simulink model "with_torque_vectoring"  (R2024b)
settings: Solver=VariableStepAuto  StartTime=0.0  StopTime=10.0  MaxStep=0.001  RelTol=1e-3
values from neighbouring files (symbols this model uses):
  c_yf = 15714    [vehicle_input_data.m]
  c_yr = 21429    [vehicle_input_data.m]
  delta = 1.04    [vehicle_input_data.m]
  dt = 0.001    [vehicle_input_data.m]
  Izz = 120    [vehicle_input_data.m]
  l_f = 0.873    [vehicle_input_data.m]
  l_r = 0.717    [vehicle_input_data.m]
  m = 356    [vehicle_input_data.m]
  VCG = 25    [vehicle_input_data.m]
libraries: slpidlib x1
settings Model: Creator=abhip  LastModifiedBy=abhip

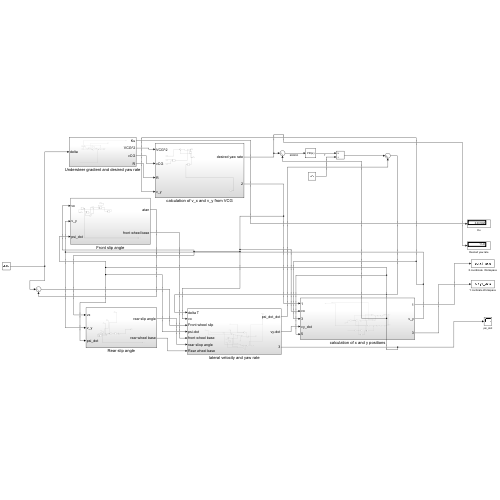
[thumbnail: Simulink's stored preview of the top-level diagram]
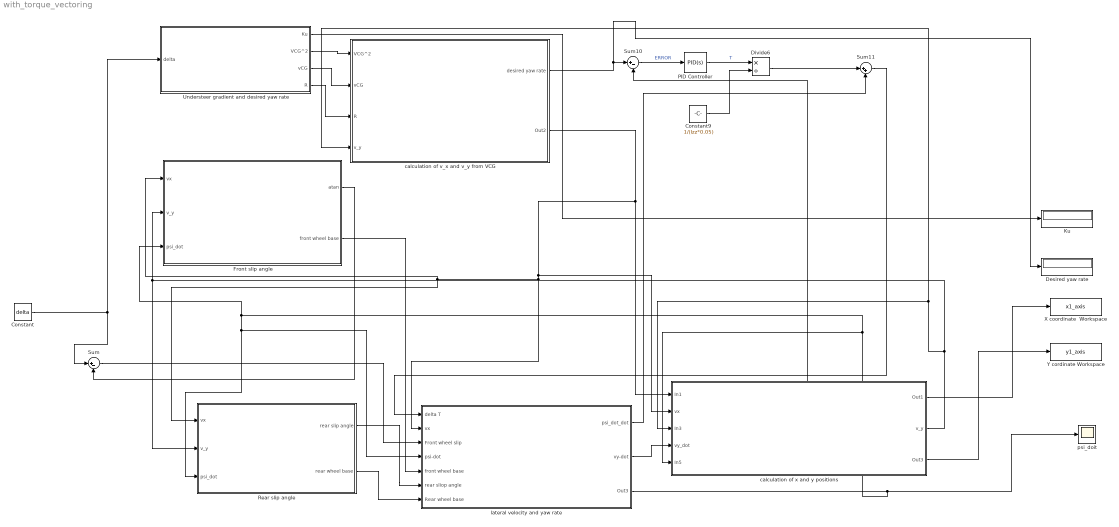
== system with_torque_vectoring ==
  Constant : Constant  Value=delta
  Constant9 : Constant  Value=1/(Izz*0.05)
  Desired yaw rate : Display
  Divide6 : Product  Inputs=*/
  Front slip angle : Subsystem
  Ku : Display
  PID Controller : slpidlib/PID Controller  Controller=PID  Form=Parallel  TimeDomain=Continuous-time  UseExternalTs=off  SampleTime=-1  IntegratorMethod=Forward Euler  FilterMethod=Forward Euler  ControllerParametersSource=internal  P=108  I=1848  UseKiTs=off  D=-0.42  UseExternalDerivativeSource=off  N=100  UseFilter=on  TunerSelectOption=Transfer Function Based (PID Tuner App)  InitialConditionSource=internal  InitialConditionForIntegrator=0  InitialConditionForFilter=0  DifferentiatorICPrevScaledInput=0  ExternalReset=none  TrackingMode=off  Kt=1  LimitOutput=off  SatLimitsSource=internal  UpperSaturationLimit=inf  LowerSaturationLimit=-inf  LinearizeAsGain=on  AntiWindupMode=none  Kb=1  LimitIntegrator=off  UpperIntegratorSaturationLimit=inf  LowerIntegratorSaturationLimit=-inf  POutMin=[]  POutMax=[]  IOutMin=[]  IOutMax=[]  DOutMin=[]  DOutMax=[]  NOutMin=[]  NOutMax=[]  SumOutMin=[]  SumOutMax=[]  SaturationOutMin=[]  SaturationOutMax=[]  PParamMin=[]  PParamMax=[]  IParamMin=[]  IParamMax=[]  DParamMin=[]  DParamMax=[]  NParamMin=[]  NParamMax=[]  KbParamMin=[]  KbParamMax=[]  KtParamMin=[]  KtParamMax=[]  KbOutMin=[]  KbOutMax=[]  KtOutMin=[]  KtOutMax=[]  IntegratorOutMin=[]  IntegratorOutMax=[]  FilterOutMin=[]  FilterOutMax=[]  SumI1OutMin=[]  SumI1OutMax=[]  SumI2OutMin=[]  SumI2OutMax=[]  SumI3OutMin=[]  SumI3OutMax=[]  SumI4OutMin=[]  SumI4OutMax=[]  SumDOutMin=[]  SumDOutMax=[]  DifferentiatorOutMin=[]  DifferentiatorOutMax=[]  FilterDiffOutCoefMin=[]  FilterDiffOutCoefMax=[]  ReciprocalOutMin=[]  ReciprocalOutMax=[]  SumDenOutMin=[]  SumDenOutMax=[]  SumNumOutMin=[]  SumNumOutMax=[]  DivideOutMin=[]  DivideOutMax=[]  UdiffTsProdOutMin=[]  UdiffTsProdOutMax=[]  NTsProdOutMin=[]  NTsProdOutMax=[]  UintegralTsProdOutMin=[]  UintegralTsProdOutMax=[]  UngainTsProdOutMin=[]  UngainTsProdOutMax=[]  ClampingZeroOutDataTypeStr=Inherit: Inherit via back propagation  ClampingZeroOutMin=[]  ClampingZeroOutMax=[]  FilterDenConstantOutDataTypeStr=Inherit: Inherit via back propagation  FilterDenConstantOutMin=[]  FilterDenConstantOutMax=[]  PCopyOutDataTypeStr=Inherit: Inherit via back propagation  PCopyOutMin=[]  PCopyOutMax=[]  NCopyOutDataTypeStr=Inherit: Inherit via back propagation  NCopyOutMin=[]  NCopyOutMax=[]  IntegratorContinuousStateAttributes=''  IntegratorStateMustResolveToSignalObject=off  IntegratorRTWStateStorageClass=Auto  FilterContinuousStateAttributes=''  FilterStateMustResolveToSignalObject=off  FilterRTWStateStorageClass=Auto  ParallelPVariant=InternalParameters  IdealPVariant=Disabled  IVariant=InternalParameters  DVariant=InternalParameters  IntegratorVariant=Continuous  SatVariant=Disabled  AWVariant=Passthrough  PCopyVariant=Disabled  TRVariant=Disabled  FdbkBlocksVariant=Forward  IdealPFdbkVariant=Disabled  SatFdbkVariant=Disabled  DerivativeFilterVariant=ContFilter  NVariant=InternalParameters  NCopyVariant=Disabled  FilterICVariant=InternalICsFilter  IntegratorICVariant=InternalICs  ExternalResetVariant=Disabled  TRSumVariant=Passthrough  SumFdbkVariant=Disabled  SumVariant=Sum_PID  TsampFilterVariant=InternalTs  TsampNgainVariant=Passthrough  TsampIntegralVariant=Disabled_SignalSpec  ExternalSaturationOutDataTypeStr=Inherit: Same as second input  DerivativeSourceVariant=ErrorSignal  PreIntVariant=InternalPreInt
  Rear slip angle : Subsystem
  Sum : Sum  Inputs=|+-
  Sum10 : Sum  Inputs=|+-
  Sum11 : Sum  Inputs=|++
  Understeer gradient and desired yaw rate : Subsystem
  X coordinate  Workspace : ToWorkspace  VariableName=x1_axis  SampleTime=-1
  Y cordinate Workspace : ToWorkspace  VariableName=y1_axis  SampleTime=-1
  calculation of v_x and v_y from VCG : Subsystem
  calculation of x and y positions : Subsystem
  "lateral velocity and yaw rate " : Subsystem
  psi_doit : Scope
  wires:
  Constant/1 -> Understeer gradient and desired yaw rate/1(delta), Sum/1
  Sum10/1 -> PID Controller/1  "ERROR"
  PID Controller/1 -> Divide6/1  "T"
  Constant9/1 -> Divide6/2
  Divide6/1 -> Sum11/1
  Front slip angle/1(atan) -> Sum/2
  Understeer gradient and desired yaw rate/1(Ku) -> Ku/1
  calculation of v_x and v_y from VCG/2(Out2) -> calculation of x and y positions/1(In1), Front slip angle/1(vx), Rear slip angle/1(vx), "lateral velocity and yaw rate "/2(vx), calculation of x and y positions/2(vx)
  calculation of v_x and v_y from VCG/1(desired yaw rate) -> Desired yaw rate/1, Sum10/1
  Understeer gradient and desired yaw rate/2(VCG^2) -> calculation of v_x and v_y from VCG/1(VCG^2)
  Understeer gradient and desired yaw rate/3(vCG) -> calculation of v_x and v_y from VCG/2(vCG)
  Understeer gradient and desired yaw rate/4(R) -> calculation of v_x and v_y from VCG/3(R)
  "lateral velocity and yaw rate "/3(Out3) -> psi_doit/1, "lateral velocity and yaw rate "/4(psi-dot), Rear slip angle/3(psi_dot), Front slip angle/3(psi_dot), calculation of x and y positions/5(In5), Sum10/2
  Sum11/1 -> "lateral velocity and yaw rate "/1(delta T)
  Sum/1 -> "lateral velocity and yaw rate "/3(Front wheel slip)
  Front slip angle/2(front wheel base) -> "lateral velocity and yaw rate "/5(front wheel base)
  Rear slip angle/1(rear slip angle) -> "lateral velocity and yaw rate "/6(rear sliop angle)
  Rear slip angle/2(rear wheel base) -> "lateral velocity and yaw rate "/7(Rear wheel base)
  "lateral velocity and yaw rate "/1(psi_dot_dot) -> Sum11/2
  calculation of x and y positions/3(Out3) -> Y cordinate Workspace/1
  calculation of x and y positions/2(v_y) -> calculation of v_x and v_y from VCG/4(v_y), calculation of x and y positions/3(In3), Rear slip angle/2(v_y), Front slip angle/2(v_y)
  calculation of x and y positions/1(Out1) -> X coordinate  Workspace/1
  "lateral velocity and yaw rate "/2(vy-dot) -> calculation of x and y positions/4(vy_dot)

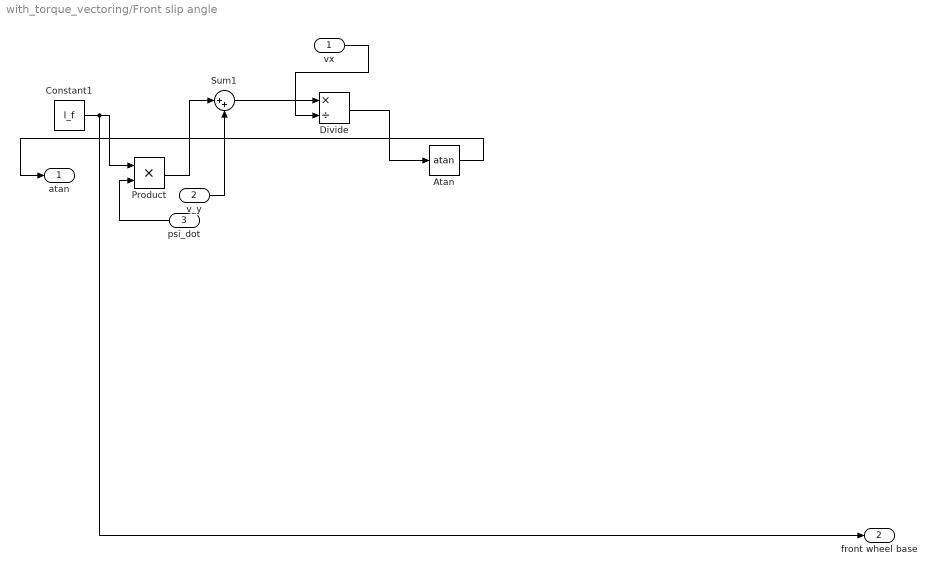
== system with_torque_vectoring/Front slip angle ==
  vx : Inport
  v_y : Inport  Port=2
  psi_dot : Inport  Port=3
  Atan : Trigonometry  Operator=atan
  Constant1 : Constant  Value=l_f
  Divide : Product  Inputs=*/
  Product : Product
  Sum1 : Sum  Inputs=|++
  atan : Outport
  front wheel base : Outport  Port=2
  wires:
  Divide/1 -> Atan/1
  Sum1/1 -> Divide/1
  Atan/1 -> atan/1
  psi_dot/1 -> Product/2
  Constant1/1 -> front wheel base/1, Product/1
  Product/1 -> Sum1/1
  vx/1 -> Divide/2
  v_y/1 -> Sum1/2

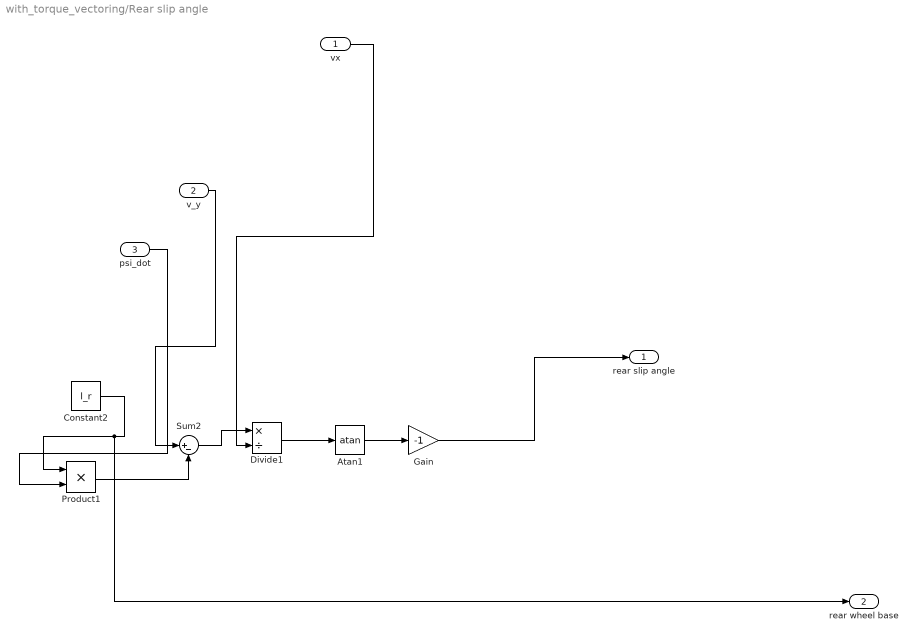
== system with_torque_vectoring/Rear slip angle ==
  vx : Inport
  v_y : Inport  Port=2
  psi_dot : Inport  Port=3
  Atan1 : Trigonometry  Operator=atan
  Constant2 : Constant  Value=l_r
  Divide1 : Product  Inputs=*/
  Gain : Gain  Gain=-1
  Product1 : Product
  Sum2 : Sum  Inputs=|+-
  rear slip angle : Outport
  rear wheel base : Outport  Port=2
  wires:
  Atan1/1 -> Gain/1
  Constant2/1 -> rear wheel base/1, Product1/1
  Sum2/1 -> Divide1/1
  Product1/1 -> Sum2/2
  vx/1 -> Divide1/2
  v_y/1 -> Sum2/1
  Divide1/1 -> Atan1/1
  Gain/1 -> rear slip angle/1
  psi_dot/1 -> Product1/2

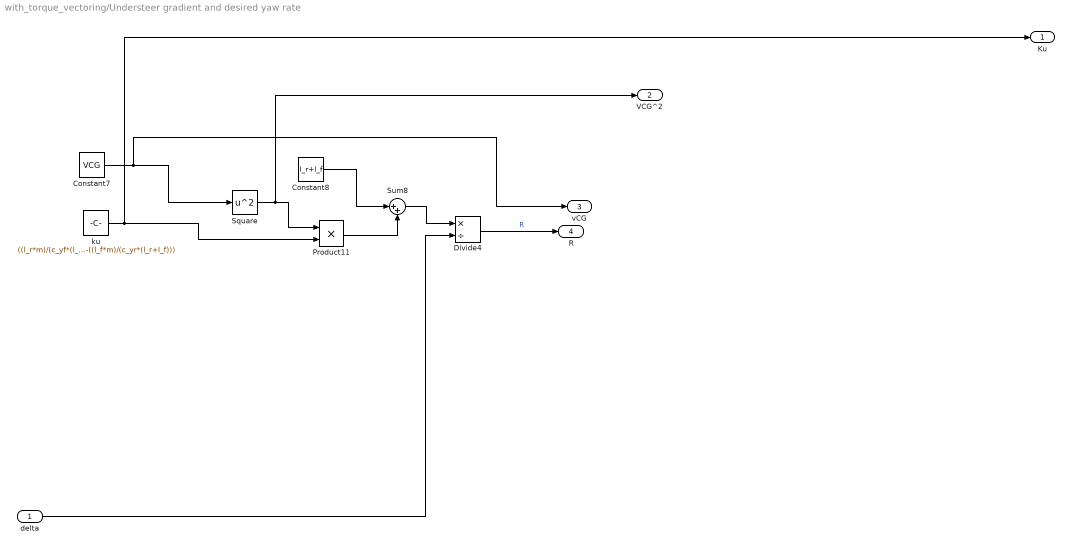
== system with_torque_vectoring/Understeer gradient and desired yaw rate ==
  delta : Inport
  Constant7 : Constant  Value=VCG
  Constant8 : Constant  Value=l_r+l_f
  Divide4 : Product  Inputs=*/
  Product11 : Product
  Square : Math  Operator=square
  Sum8 : Sum  Inputs=|++
  ku : Constant  Value=((l_r*m)/(c_yf*(l_r+l_f)))-((l_f*m)/(c_yr*(l_r+l_f)))
  Ku : Outport
  VCG^2 : Outport  Port=2
  vCG : Outport  Port=3
  R : Outport  Port=4
  wires:
  Product11/1 -> Sum8/2
  ku/1 -> Ku/1, Product11/2
  Constant7/1 -> vCG/1, Square/1
  Square/1 -> VCG^2/1, Product11/1
  delta/1 -> Divide4/2
  Sum8/1 -> Divide4/1
  Constant8/1 -> Sum8/1
  Divide4/1 -> R/1  "R"

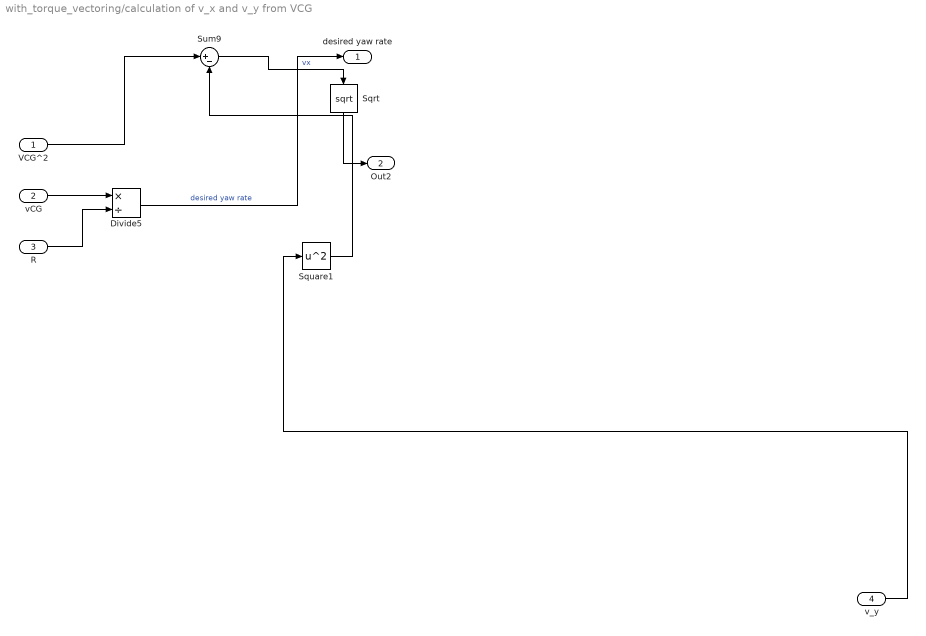
== system with_torque_vectoring/calculation of v_x and v_y from VCG ==
  VCG^2 : Inport
  vCG : Inport  Port=2
  R : Inport  Port=3
  v_y : Inport  Port=4
  Divide5 : Product  Inputs=*/
  Sqrt : Sqrt
  Square1 : Math  Operator=square
  Sum9 : Sum  Inputs=|+-
  desired yaw rate : Outport
  Out2 : Outport  Port=2
  wires:
  Sqrt/1 -> Out2/1
  Divide5/1 -> desired yaw rate/1  "desired yaw rate"
  Square1/1 -> Sum9/2
  vCG/1 -> Divide5/1
  R/1 -> Divide5/2
  v_y/1 -> Square1/1
  VCG^2/1 -> Sum9/1
  Sum9/1 -> Sqrt/1  "vx"

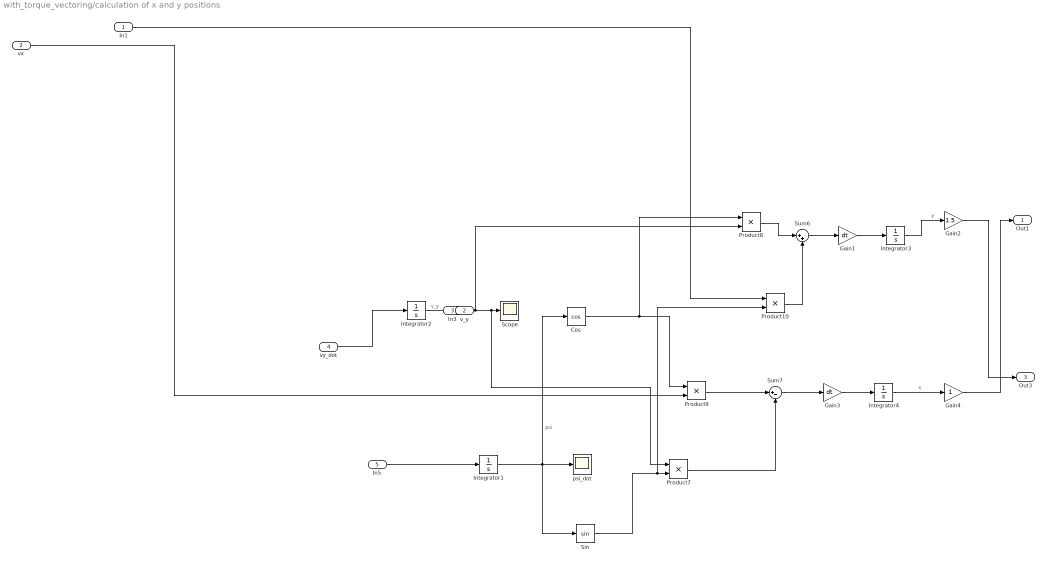
== system with_torque_vectoring/calculation of x and y positions ==
  In1 : Inport
  vx : Inport  Port=2
  In3 : Inport  Port=3
  vy_dot : Inport  Port=4
  In5 : Inport  Port=5
  Cos : Trigonometry  Operator=cos
  Gain1 : Gain  Gain=dt
  Gain2 : Gain  Gain=1.5
  Gain3 : Gain  Gain=dt
  Gain4 : Gain
  Integrator{1..4} (4 alike) : Integrator
  Product{7..10} (4 alike) : Product
  Scope : Scope
  Sin : Trigonometry
  Sum6 : Sum  Inputs=|++
  Sum7 : Sum  Inputs=|+-
  psi_dot : Scope
  Out1 : Outport
  v_y : Outport  Port=2
  Out3 : Outport  Port=3
  wires:
  Product7/1 -> Sum7/2
  Integrator1/1 -> Cos/1, Sin/1, psi_dot/1  "psi"
  Cos/1 -> Product8/1, Product9/1
  Sum6/1 -> Gain1/1
  Product9/1 -> Sum7/1
  In3/1 -> Product8/2, Product7/1, Scope/1
  Gain1/1 -> Integrator3/1
  Integrator3/1 -> Gain2/1  "y"
  Sin/1 -> Product10/2, Product7/2
  Product10/1 -> Sum6/2
  Sum7/1 -> Gain3/1
  In1/1 -> Product10/1
  Integrator4/1 -> Gain4/1  "x"
  Gain3/1 -> Integrator4/1
  Gain4/1 -> Out1/1
  Product8/1 -> Sum6/1
  vx/1 -> Product9/2
  Gain2/1 -> Out3/1
  Integrator2/1 -> v_y/1  "v_y"
  In5/1 -> Integrator1/1
  vy_dot/1 -> Integrator2/1

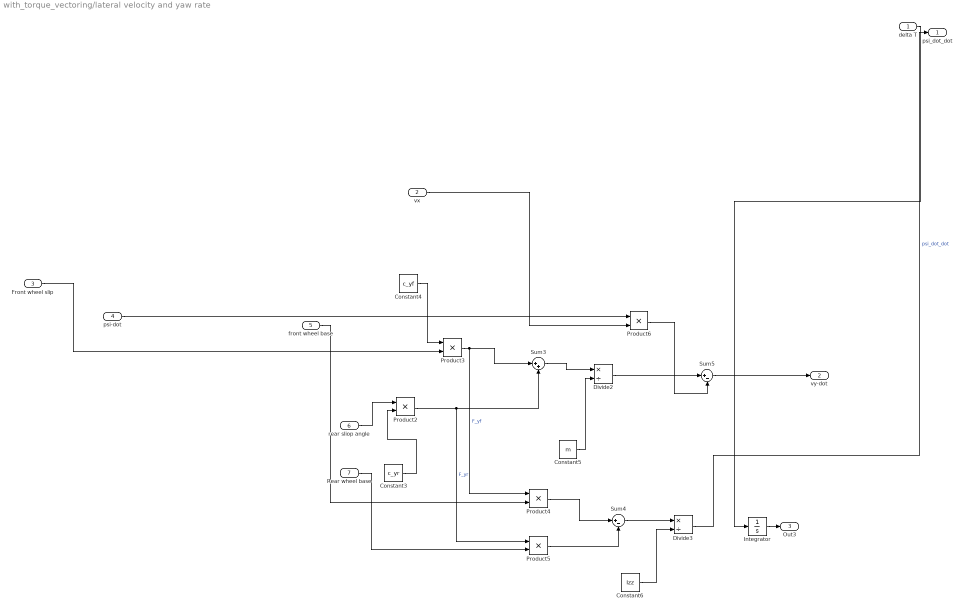
== system with_torque_vectoring/lateral velocity and yaw rate  ==
  delta T : Inport
  vx : Inport  Port=2
  Front wheel slip : Inport  Port=3
  psi-dot : Inport  Port=4
  front wheel base : Inport  Port=5
  rear sliop angle : Inport  Port=6
  Rear wheel base : Inport  Port=7
  Constant3 : Constant  Value=c_yr
  Constant4 : Constant  Value=c_yf
  Constant5 : Constant  Value=m
  Constant6 : Constant  Value=Izz
  Divide2 : Product  Inputs=*/
  Divide3 : Product  Inputs=*/
  Integrator : Integrator
  Product{2..6} (5 alike) : Product
  Sum3 : Sum  Inputs=|++
  Sum4 : Sum  Inputs=|+-
  Sum5 : Sum  Inputs=|+-
  psi_dot_dot : Outport
  vy-dot : Outport  Port=2
  Out3 : Outport  Port=3
  wires:
  Constant6/1 -> Divide3/2
  delta T/1 -> Integrator/1
  Constant3/1 -> Product2/2
  Product3/1 -> Product4/1, Sum3/1  "F_yf"
  Product6/1 -> Sum5/2
  Constant5/1 -> Divide2/2
  Rear wheel base/1 -> Product5/2
  Sum3/1 -> Divide2/1
  Product2/1 -> Product5/1, Sum3/2  "F_yr"
  Divide2/1 -> Sum5/1
  Product5/1 -> Sum4/2
  Constant4/1 -> Product3/1
  front wheel base/1 -> Product4/2
  Sum4/1 -> Divide3/1
  Product4/1 -> Sum4/1
  vx/1 -> Product6/2
  rear sliop angle/1 -> Product2/1
  Front wheel slip/1 -> Product3/2
  Integrator/1 -> Out3/1
  psi-dot/1 -> Product6/1
  Sum5/1 -> vy-dot/1
  Divide3/1 -> psi_dot_dot/1  "psi_dot_dot"
